simulink model "bee2_complex_corr"  (Simulink 7.0)
settings: Solver=ode45  StartTime=0.0  StopTime=10.0  RelTol=1e-3
undefined symbols (not defined in the file or in its folder): BEE2_usr
libraries: xbsIndex_r4 x279, xps_library x61, casper_library_misc x18
(part 1 of 4)
settings Model: Creator=Rurik A Primiani  LastModifiedBy=mdexter

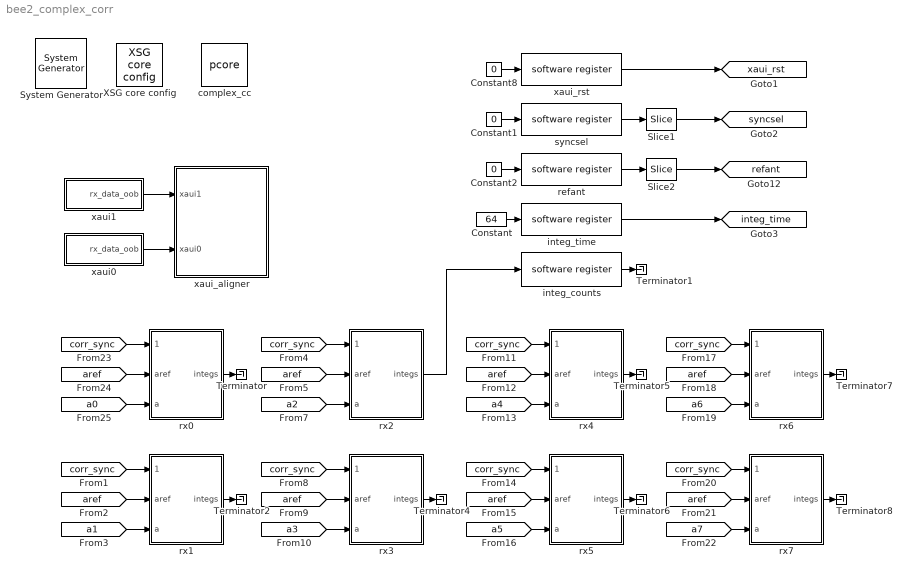
== system bee2_complex_corr ==
  " System Generator" : xbsIndex_r4/ System Generator  Tag=genX  SystemSampleTime=-1  xilinxfamily=virtex2p  part=xc2vp70  speed=-7  package=ff1704  synthesis_tool=XST  clock_wrapper=Clock Enables  directory=./bee2_complex_corr/sysgen  testbench=off  simulink_period=1  sysclk_period=3.9063  dcm_input_clock_period=100  incr_netlist=off  trim_vbits=Everywhere in SubSystem  dbl_ovrd=According to Block Masks  core_generation=According to Block Masks  run_coregen=off  deprecated_control=off  eval_field=0  block_type=sysgen
      settings: block_version=10.1.3
  Constant : Constant  Value=64
  Constant1 : Constant  Value=0
  Constant2 : Constant  Value=0
  Constant8 : Constant  Value=0
  Slice1 : xbsIndex_r4/Slice  nbits=2  boolean_output=off  mode=Lower Bit Location + Width  bit1=0  base1=MSB of Input  bit0=0  base0=LSB of Input  dbl_ovrd=off  block_type=slice
      settings: infoedit="Extracts a given range of bits from each input sample and presents it at the output.  The output type is ordinarily unsigned with binary point at zero, but can be Boolean when the slice is one bit wide.<P><P>Hardware notes: In hardware this block costs nothing."  block_version=10.1.3
  Slice2 : xbsIndex_r4/Slice  nbits=3  boolean_output=off  mode=Lower Bit Location + Width  bit1=0  base1=MSB of Input  bit0=0  base0=LSB of Input  dbl_ovrd=off  block_type=slice
      settings: infoedit="Extracts a given range of bits from each input sample and presents it at the output.  The output type is ordinarily unsigned with binary point at zero, but can be Boolean when the slice is one bit wide.<P><P>Hardware notes: In hardware this block costs nothing."  block_version=10.1.3
  Terminator{,1..2,4..8} (8 alike) : Terminator
  XSG core config : xps_library/XSG core config  Tag=xps:xsg  SystemSampleTime=-1  hw_sys=BEE2_usr  ibob_linux=off  clk_src=usr_clk2x  iBOB_clk_src=sys_clk  BEE2_ctrl_clk_src=sys_clk  BEE2_usr_clk_src=usr_clk2x  ROACH_clk_src=sys_clk  CORR_clk_src=sys_clk  gpio_clk_io_group=iBOB:sma  gpio_clk_bit_index=0  clk_rate=256  sample_period=1  synthesis_tool=XST  mpc_type=powerpc405
  complex_cc : xps_library/pcore  Tag=xps:pcore  SystemSampleTime=-1  pcore_path=complex_cc_core/complex_cc_core.ngc
  integ_counts : xps_library/software register  Tag=xps:sw_reg  SystemSampleTime=-1  io_dir=To Processor  arith_type=Unsigned  bitwidth=32  bin_pt=0  sample_period=1  gw_name=bee2_complex_corr_integ_counts_user_data_in
      link override convert: arith_type=Unsigned  n_bits=32  bin_pt=0
  integ_time : xps_library/software register  Tag=xps:sw_reg  SystemSampleTime=-1  io_dir=From Processor  arith_type=Unsigned  bitwidth=32  bin_pt=0  sample_period=1  gw_name=bee2_complex_corr_integ_time_user_data_out
      link override bee2_complex_corr_0x0_integ_time_user_data_out: arith_type=Unsigned  n_bits=32  bin_pt=0  period=1
      link override bee2_complex_corr_corr00_integ_time_user_data_out: arith_type=Unsigned  n_bits=32  bin_pt=0  period=1
      link override bee2_complex_corr_corr01_integ_time_user_data_out: arith_type=Unsigned  n_bits=32  bin_pt=0  period=1
      link override bee2_complex_corr_integ_time_user_data_out: arith_type=Unsigned  n_bits=32  bin_pt=0  period=1
      link override correlator_2bit_bee2_integ_time_user_data_out: arith_type=Unsigned  n_bits=32  bin_pt=0  period=1
      link override correlator_2bit_bee2_x2_integ_time_user_data_out: arith_type=Unsigned  n_bits=32  bin_pt=0  period=1
      link override correlator_2bit_ibob_integ_time_user_data_out: arith_type=Unsigned  n_bits=32  bin_pt=0  period=1
      link override dbe_xaui_corr_corr_integ_time_user_data_out: arith_type=Unsigned  n_bits=32  bin_pt=0  period=1
      link override dbe_xaui_corr_corr_integ_user_data_out: arith_type=Unsigned  n_bits=32  bin_pt=0  period=1
      link override dbe_xaui_corr_new_corr_integ_user_data_out: arith_type=Unsigned  n_bits=32  bin_pt=0  period=1
  refant : xps_library/software register  Tag=xps:sw_reg  SystemSampleTime=-1  io_dir=From Processor  arith_type=Unsigned  bitwidth=32  bin_pt=0  sample_period=1  gw_name=bee2_complex_corr_refant_user_data_out
      link override bee2_complex_corr_corr_rst_user_data_out: arith_type=Unsigned  n_bits=32  bin_pt=0  period=1
      link override bee2_complex_corr_refant_user_data_out: arith_type=Unsigned  n_bits=32  bin_pt=0  period=1
      link override correlator_2bit_bee2_integ_time_user_data_out: arith_type=Unsigned  n_bits=32  bin_pt=0  period=1
      link override correlator_2bit_bee2_x2_integ_time_user_data_out: arith_type=Unsigned  n_bits=32  bin_pt=0  period=1
      link override correlator_2bit_ibob_integ_time_user_data_out: arith_type=Unsigned  n_bits=32  bin_pt=0  period=1
      link override dbe_xaui_corr_corr_integ_user_data_out: arith_type=Unsigned  n_bits=32  bin_pt=0  period=1
      link override dbe_xaui_corr_corr_reset_user_data_out: arith_type=Unsigned  n_bits=32  bin_pt=0  period=1
      link override dbe_xaui_corr_new_corr_integ_user_data_out: arith_type=Unsigned  n_bits=32  bin_pt=0  period=1
  rx0 : Subsystem
  rx1 : Subsystem
  rx2 : Subsystem
  rx3 : Subsystem
  rx4 : Subsystem
  rx5 : Subsystem
  rx6 : Subsystem
  rx7 : Subsystem
  syncsel : xps_library/software register  Tag=xps:sw_reg  SystemSampleTime=-1  io_dir=From Processor  arith_type=Unsigned  bitwidth=32  bin_pt=0  sample_period=1  gw_name=bee2_complex_corr_syncsel_user_data_out
      link override bee2_complex_corr_corr_rst_user_data_out: arith_type=Unsigned  n_bits=32  bin_pt=0  period=1
      link override bee2_complex_corr_syncsel_user_data_out: arith_type=Unsigned  n_bits=32  bin_pt=0  period=1
      link override correlator_2bit_bee2_integ_time_user_data_out: arith_type=Unsigned  n_bits=32  bin_pt=0  period=1
      link override correlator_2bit_bee2_x2_integ_time_user_data_out: arith_type=Unsigned  n_bits=32  bin_pt=0  period=1
      link override correlator_2bit_ibob_integ_time_user_data_out: arith_type=Unsigned  n_bits=32  bin_pt=0  period=1
      link override dbe_xaui_corr_corr_integ_user_data_out: arith_type=Unsigned  n_bits=32  bin_pt=0  period=1
      link override dbe_xaui_corr_corr_reset_user_data_out: arith_type=Unsigned  n_bits=32  bin_pt=0  period=1
      link override dbe_xaui_corr_new_corr_integ_user_data_out: arith_type=Unsigned  n_bits=32  bin_pt=0  period=1
  xaui0 : Subsystem
  xaui1 : Subsystem
  xaui_aligner : Subsystem
  xaui_rst : xps_library/software register  Tag=xps:sw_reg  SystemSampleTime=-1  io_dir=From Processor  arith_type=Unsigned  bitwidth=32  bin_pt=0  sample_period=1  gw_name=bee2_complex_corr_xaui_rst_user_data_out
      link override bee2_complex_corr_xaui_rst_user_data_out: arith_type=Unsigned  n_bits=32  bin_pt=0  period=1
      link override dbe_xaui_corr_xaui_rst_user_data_out: arith_type=Unsigned  n_bits=32  bin_pt=0  period=1
      link override dbe_xaui_xaui_rst_user_data_out: arith_type=Unsigned  n_bits=32  bin_pt=0  period=1
      link override xaui_rx_reset_user_data_out: arith_type=Unsigned  n_bits=32  bin_pt=0  period=1
  tag scope: integ_time=global, refant=global, syncsel=global, xaui_rst=global
  wires:
  xaui1/1(rx_data_oob) -> xaui_aligner/1(xaui1)
  xaui0/1(rx_data_oob) -> xaui_aligner/2(xaui0)
  xaui_rst/1 -> [xaui_rst]
  Constant8/1 -> xaui_rst/1
  syncsel/1 -> Slice1/1
  Slice1/1 -> [syncsel]
  Constant1/1 -> syncsel/1
  [corr_sync] -> rx1/1(sync_in)
  [aref] -> rx1/2(aref)
  [a1] -> rx1/3(a)
  [corr_sync] -> rx2/1(sync_in)
  [aref] -> rx2/2(aref)
  [a2] -> rx2/3(a)
  [corr_sync] -> rx3/1(sync_in)
  [aref] -> rx3/2(aref)
  [a3] -> rx3/3(a)
  [corr_sync] -> rx4/1(sync_in)
  [aref] -> rx4/2(aref)
  [a4] -> rx4/3(a)
  [corr_sync] -> rx5/1(sync_in)
  [aref] -> rx5/2(aref)
  [a5] -> rx5/3(a)
  [corr_sync] -> rx6/1(sync_in)
  [aref] -> rx6/2(aref)
  [a6] -> rx6/3(a)
  [corr_sync] -> rx7/1(sync_in)
  [aref] -> rx7/2(aref)
  [a7] -> rx7/3(a)
  [corr_sync] -> rx0/1(sync_in)
  [aref] -> rx0/2(aref)
  [a0] -> rx0/3(a)
  refant/1 -> Slice2/1
  Slice2/1 -> [refant]
  Constant2/1 -> refant/1
  integ_time/1 -> [integ_time]
  rx0/1(integs) -> Terminator/1
  integ_counts/1 -> Terminator1/1
  Constant/1 -> integ_time/1
  rx1/1(integs) -> Terminator2/1
  rx3/1(integs) -> Terminator4/1
  rx4/1(integs) -> Terminator5/1
  rx5/1(integs) -> Terminator6/1
  rx6/1(integs) -> Terminator7/1
  rx7/1(integs) -> Terminator8/1
  rx2/1(integs) -> integ_counts/1

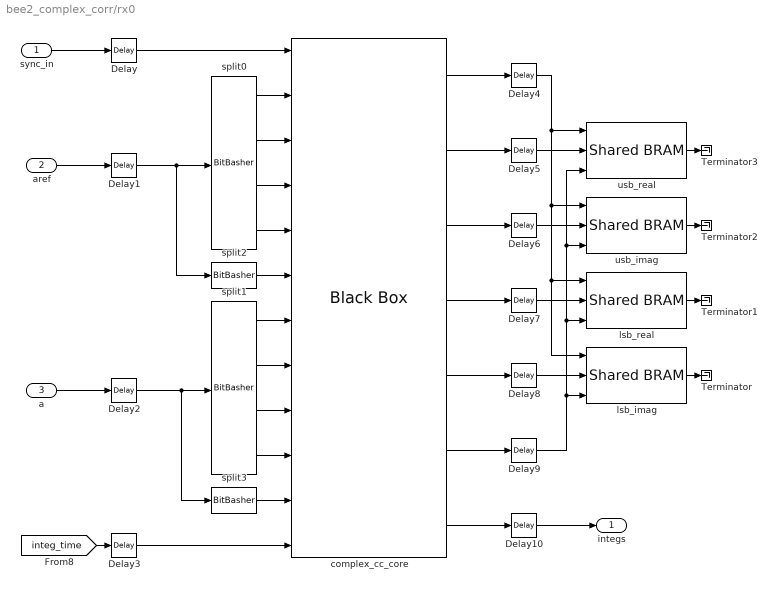
== system bee2_complex_corr/rx0 ==
  sync_in : Inport  OutDataType=sfix(16)  OutScaling=2^0
  aref : Inport  Port=2  OutDataType=sfix(16)  OutScaling=2^0
  a : Inport  Port=3  OutDataType=sfix(16)  OutScaling=2^0
  Delay{,1..10} (11 alike) : xbsIndex_r4/Delay  en=off  latency=1  dbl_ovrd=off  reg_retiming=off  block_type=delay
  Terminator{,1..3} (4 alike) : Terminator
  complex_cc_core : xbsIndex_r4/Black Box  init_code=complex_cc_core_config  sim_method=Inactive  block_type=blackbox2
      settings: infoedit="Incorporates black box HDL and simulation model into a System Generator design.<P><P>You must supply a Black Box with certain information about the HDL component you would like to bring into System Generator. This information is provided through a Matlab function.<P><P>When \"Simulation mode\" is set to \"Inactive\", you will typically want to provide a separate simulation model by using a Simulation Multiplexer.<P>When \"Simulation mode\" is set to \"External co-simulator\", you must include a ModelSim block in the design."  block_version=10.1.3
  lsb_imag : xps_library/Shared BRAM  Tag=xps:bram  SystemSampleTime=-1  arith_type="Signed  (2's comp)"  addr_width=11  data_width=32  data_bin_pt=0  init_vals=0  sample_rate=1
      link override bee2_complex_corr_0x0_func_real_data_out: arith_type="Signed  (2's comp)"
      link override bee2_complex_corr_corr00_func_real_data_out: arith_type="Signed  (2's comp)"
      link override bee2_complex_corr_corr01_func_real_data_out: arith_type="Signed  (2's comp)"
      link override bee2_complex_corr_rx0_lsb_imag_data_out: arith_type="Signed  (2's comp)"
      link override convert_din: arith_type="Signed  (2's comp)"
      link override correlator_2bit_bee2_output_corr0_data_out: arith_type=Unsigned
      link override correlator_2bit_bee2_x2_output_corr01_data_out: arith_type=Unsigned
      link override correlator_2bit_bee2_x2_output_corr0_data_out: arith_type=Unsigned
      link override correlator_2bit_ibob_output_corr0_data_out: arith_type=Unsigned
      link override cross_correlator_test_corr_out_data_out: arith_type="Signed  (2's comp)"
      link override cross_correlator_test_input_data1_data_out: arith_type=Unsigned
      link override dbe_xaui_corr_corr_func_data_out: arith_type="Signed  (2's comp)"
      link override dbe_xaui_corr_new_xaui_summer_summer_output_corr_data_out: arith_type="Signed  (2's comp)"
      link override dbe_xaui_corr_xaui_summer_summer_output_corr_data_out: arith_type="Signed  (2's comp)"
      link override mem/sim_data_in: arith_type="Signed  (2's comp)"
  lsb_real : xps_library/Shared BRAM  Tag=xps:bram  SystemSampleTime=-1  arith_type="Signed  (2's comp)"  addr_width=11  data_width=32  data_bin_pt=0  init_vals=0  sample_rate=1
      link override bee2_complex_corr_0x0_func_real_data_out: arith_type="Signed  (2's comp)"
      link override bee2_complex_corr_corr00_func_real_data_out: arith_type="Signed  (2's comp)"
      link override bee2_complex_corr_corr01_func_real_data_out: arith_type="Signed  (2's comp)"
      link override bee2_complex_corr_rx0_lsb_real_data_out: arith_type="Signed  (2's comp)"
      link override convert_din: arith_type="Signed  (2's comp)"
      link override correlator_2bit_bee2_output_corr0_data_out: arith_type=Unsigned
      link override correlator_2bit_bee2_x2_output_corr01_data_out: arith_type=Unsigned
      link override correlator_2bit_bee2_x2_output_corr0_data_out: arith_type=Unsigned
      link override correlator_2bit_ibob_output_corr0_data_out: arith_type=Unsigned
      link override cross_correlator_test_corr_out_data_out: arith_type="Signed  (2's comp)"
      link override cross_correlator_test_input_data1_data_out: arith_type=Unsigned
      link override dbe_xaui_corr_corr_func_data_out: arith_type="Signed  (2's comp)"
      link override dbe_xaui_corr_new_xaui_summer_summer_output_corr_data_out: arith_type="Signed  (2's comp)"
      link override dbe_xaui_corr_xaui_summer_summer_output_corr_data_out: arith_type="Signed  (2's comp)"
      link override mem/sim_data_in: arith_type="Signed  (2's comp)"
  split0 : xbsIndex_r4/BitBasher  bitexpr=|  display_expr=off  sr_1=1  arith_type1=Unsigned  bin_pt1=0  sr_2=2  arith_type2=Unsigned  bin_pt2=0  sr_3=3  arith_type3=Unsigned  bin_pt3=0  sr_4=4  arith_type4=Unsigned  bin_pt4=0  dbl_ovrd=off  block_type=bitbasher
      | <html><head><meta name="qrichtext" content="1" /><style type="text/css">
      | p, li { white-space: pre-wrap; }
      | </style></head><body style=" font-family:'MS Shell Dlg 2'; font-size:8.25pt; font-weight:400; font-style:normal;">
      | <p style=" margin-top:0px; margin-bottom:0px; margin-left:0px; margin-right:0px; -qt-block-indent:0; text-indent:0px; font-size:8pt;">r0={a[8:7]}<br />i0={a[6:5]}<br /><span style=" font-family:'MS Shell Dlg';">r1={a[4:3]}<br />i1={a[2:1]}</span></p></body></html>
      settings: block_version=10.1.3
  split1 : xbsIndex_r4/BitBasher  bitexpr=|  display_expr=off  sr_1=1  arith_type1=Unsigned  bin_pt1=0  sr_2=2  arith_type2=Unsigned  bin_pt2=0  sr_3=3  arith_type3=Unsigned  bin_pt3=0  sr_4=4  arith_type4=Unsigned  bin_pt4=0  dbl_ovrd=off  block_type=bitbasher
      | <html><head><meta name="qrichtext" content="1" /><style type="text/css">
      | p, li { white-space: pre-wrap; }
      | </style></head><body style=" font-family:'MS Shell Dlg 2'; font-size:8.25pt; font-weight:400; font-style:normal;">
      | <p style=" margin-top:0px; margin-bottom:0px; margin-left:0px; margin-right:0px; -qt-block-indent:0; text-indent:0px; font-size:8pt;">r0={a[8:7]}<br />i0={a[6:5]}<br /><span style=" font-family:'MS Shell Dlg';">r1={a[4:3]}<br />i1={a[2:1]}</span></p></body></html>
      settings: block_version=10.1.3
  split2 : xbsIndex_r4/BitBasher  bitexpr=|  display_expr=off  sr_1=1  arith_type1=Unsigned  bin_pt1=0  sr_2=2  arith_type2=Unsigned  bin_pt2=0  sr_3=3  arith_type3=Unsigned  bin_pt3=0  sr_4=4  arith_type4=Unsigned  bin_pt4=0  dbl_ovrd=off  block_type=bitbasher
      | <html><head><meta name="qrichtext" content="1" /><style type="text/css">
      | p, li { white-space: pre-wrap; }
      | </style></head><body style=" font-family:'MS Shell Dlg 2'; font-size:8.25pt; font-weight:400; font-style:normal;">
      | <p style=" margin-top:0px; margin-bottom:0px; margin-left:0px; margin-right:0px; -qt-block-indent:0; text-indent:0px; font-size:8pt;"><span style=" font-family:'MS Shell Dlg';">w={a[0]}</span></p></body></html>
      settings: block_version=10.1.3
  split3 : xbsIndex_r4/BitBasher  bitexpr=|  display_expr=off  sr_1=1  arith_type1=Unsigned  bin_pt1=0  sr_2=2  arith_type2=Unsigned  bin_pt2=0  sr_3=3  arith_type3=Unsigned  bin_pt3=0  sr_4=4  arith_type4=Unsigned  bin_pt4=0  dbl_ovrd=off  block_type=bitbasher
      | <html><head><meta name="qrichtext" content="1" /><style type="text/css">
      | p, li { white-space: pre-wrap; }
      | </style></head><body style=" font-family:'MS Shell Dlg 2'; font-size:8.25pt; font-weight:400; font-style:normal;">
      | <p style=" margin-top:0px; margin-bottom:0px; margin-left:0px; margin-right:0px; -qt-block-indent:0; text-indent:0px; font-size:8pt;"><span style=" font-family:'MS Shell Dlg';">w={a[0]}</span></p></body></html>
      settings: block_version=10.1.3
  usb_imag : xps_library/Shared BRAM  Tag=xps:bram  SystemSampleTime=-1  arith_type="Signed  (2's comp)"  addr_width=11  data_width=32  data_bin_pt=0  init_vals=0  sample_rate=1
      link override bee2_complex_corr_0x0_func_real_data_out: arith_type="Signed  (2's comp)"
      link override bee2_complex_corr_corr00_func_real_data_out: arith_type="Signed  (2's comp)"
      link override bee2_complex_corr_corr01_func_real_data_out: arith_type="Signed  (2's comp)"
      link override bee2_complex_corr_rx0_usb_imag_data_out: arith_type="Signed  (2's comp)"
      link override convert_din: arith_type="Signed  (2's comp)"
      link override correlator_2bit_bee2_output_corr0_data_out: arith_type=Unsigned
      link override correlator_2bit_bee2_x2_output_corr01_data_out: arith_type=Unsigned
      link override correlator_2bit_bee2_x2_output_corr0_data_out: arith_type=Unsigned
      link override correlator_2bit_ibob_output_corr0_data_out: arith_type=Unsigned
      link override cross_correlator_test_corr_out_data_out: arith_type="Signed  (2's comp)"
      link override cross_correlator_test_input_data1_data_out: arith_type=Unsigned
      link override dbe_xaui_corr_corr_func_data_out: arith_type="Signed  (2's comp)"
      link override dbe_xaui_corr_new_xaui_summer_summer_output_corr_data_out: arith_type="Signed  (2's comp)"
      link override dbe_xaui_corr_xaui_summer_summer_output_corr_data_out: arith_type="Signed  (2's comp)"
      link override mem/sim_data_in: arith_type="Signed  (2's comp)"
  usb_real : xps_library/Shared BRAM  Tag=xps:bram  SystemSampleTime=-1  arith_type="Signed  (2's comp)"  addr_width=11  data_width=32  data_bin_pt=0  init_vals=0  sample_rate=1
      link override bee2_complex_corr_0x0_func_real_data_out: arith_type="Signed  (2's comp)"
      link override bee2_complex_corr_corr00_func_real_data_out: arith_type="Signed  (2's comp)"
      link override bee2_complex_corr_corr01_func_real_data_out: arith_type="Signed  (2's comp)"
      link override bee2_complex_corr_rx0_usb_real_data_out: arith_type="Signed  (2's comp)"
      link override convert_din: arith_type="Signed  (2's comp)"
      link override correlator_2bit_bee2_output_corr0_data_out: arith_type=Unsigned
      link override correlator_2bit_bee2_x2_output_corr01_data_out: arith_type=Unsigned
      link override correlator_2bit_bee2_x2_output_corr0_data_out: arith_type=Unsigned
      link override correlator_2bit_ibob_output_corr0_data_out: arith_type=Unsigned
      link override cross_correlator_test_corr_out_data_out: arith_type="Signed  (2's comp)"
      link override cross_correlator_test_input_data1_data_out: arith_type=Unsigned
      link override dbe_xaui_corr_corr_func_data_out: arith_type="Signed  (2's comp)"
      link override dbe_xaui_corr_new_xaui_summer_summer_output_corr_data_out: arith_type="Signed  (2's comp)"
      link override dbe_xaui_corr_xaui_summer_summer_output_corr_data_out: arith_type="Signed  (2's comp)"
      link override mem/sim_data_in: arith_type="Signed  (2's comp)"
  integs : Outport  OutDataType=sfix(16)  OutScaling=2^0
  wires:
  [integ_time] -> Delay3/1
  a/1 -> Delay2/1
  aref/1 -> Delay1/1
  split0/4 -> complex_cc_core/5
  split0/3 -> complex_cc_core/4
  split0/2 -> complex_cc_core/3
  split0/1 -> complex_cc_core/2
  sync_in/1 -> Delay/1
  complex_cc_core/1 -> Delay4/1
  complex_cc_core/2 -> Delay5/1
  complex_cc_core/3 -> Delay6/1
  complex_cc_core/4 -> Delay7/1
  complex_cc_core/5 -> Delay8/1
  Delay/1 -> complex_cc_core/1
  Delay1/1 -> split0/1, split2/1
  Delay2/1 -> split1/1, split3/1
  Delay7/1 -> lsb_real/2
  Delay8/1 -> lsb_imag/2
  Delay10/1 -> integs/1
  complex_cc_core/6 -> Delay9/1
  complex_cc_core/7 -> Delay10/1
  Delay5/1 -> usb_real/2
  Delay6/1 -> usb_imag/2
  Delay3/1 -> complex_cc_core/12
  split2/1 -> complex_cc_core/6
  split1/1 -> complex_cc_core/7
  split1/2 -> complex_cc_core/8
  split1/3 -> complex_cc_core/9
  split1/4 -> complex_cc_core/10
  split3/1 -> complex_cc_core/11
  Delay4/1 -> usb_real/1, usb_imag/1, lsb_imag/1, lsb_real/1
  Delay9/1 -> usb_real/3, usb_imag/3, lsb_real/3, lsb_imag/3
  lsb_imag/1 -> Terminator/1
  lsb_real/1 -> Terminator1/1
  usb_imag/1 -> Terminator2/1
  usb_real/1 -> Terminator3/1

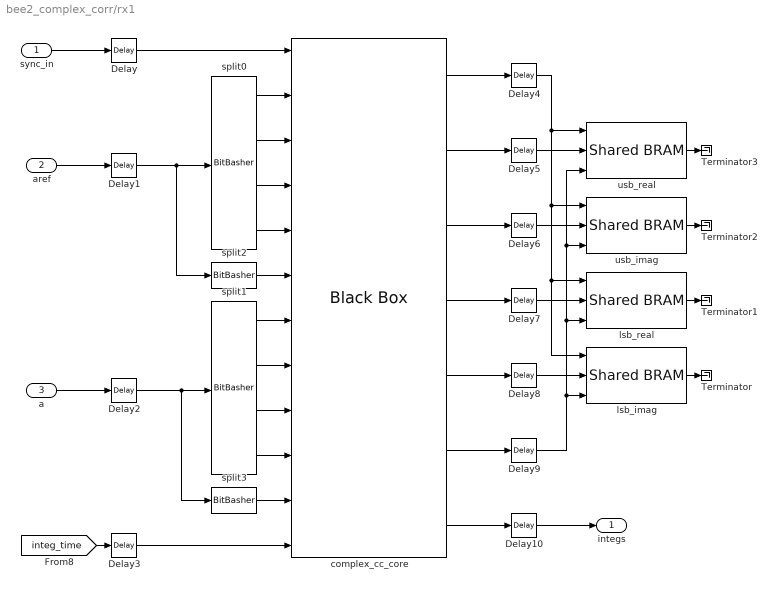
== system bee2_complex_corr/rx1 ==
  sync_in : Inport  OutDataType=sfix(16)  OutScaling=2^0
  aref : Inport  Port=2  OutDataType=sfix(16)  OutScaling=2^0
  a : Inport  Port=3  OutDataType=sfix(16)  OutScaling=2^0
  Delay{,1..10} (11 alike) : xbsIndex_r4/Delay  en=off  latency=1  dbl_ovrd=off  reg_retiming=off  block_type=delay
  Terminator{,1..3} (4 alike) : Terminator
  complex_cc_core : xbsIndex_r4/Black Box  init_code=complex_cc_core_config  sim_method=Inactive  block_type=blackbox2
      settings: infoedit="Incorporates black box HDL and simulation model into a System Generator design.<P><P>You must supply a Black Box with certain information about the HDL component you would like to bring into System Generator. This information is provided through a Matlab function.<P><P>When \"Simulation mode\" is set to \"Inactive\", you will typically want to provide a separate simulation model by using a Simulation Multiplexer.<P>When \"Simulation mode\" is set to \"External co-simulator\", you must include a ModelSim block in the design."  block_version=10.1.3
  lsb_imag : xps_library/Shared BRAM  Tag=xps:bram  SystemSampleTime=-1  arith_type="Signed  (2's comp)"  addr_width=11  data_width=32  data_bin_pt=0  init_vals=0  sample_rate=1
      link override bee2_complex_corr_0x0_func_real_data_out: arith_type="Signed  (2's comp)"
      link override bee2_complex_corr_corr00_func_real_data_out: arith_type="Signed  (2's comp)"
      link override bee2_complex_corr_corr01_func_real_data_out: arith_type="Signed  (2's comp)"
      link override bee2_complex_corr_rx1_lsb_imag_data_out: arith_type="Signed  (2's comp)"
      link override convert_din: arith_type="Signed  (2's comp)"
      link override correlator_2bit_bee2_output_corr0_data_out: arith_type=Unsigned
      link override correlator_2bit_bee2_x2_output_corr01_data_out: arith_type=Unsigned
      link override correlator_2bit_bee2_x2_output_corr0_data_out: arith_type=Unsigned
      link override correlator_2bit_ibob_output_corr0_data_out: arith_type=Unsigned
      link override cross_correlator_test_corr_out_data_out: arith_type="Signed  (2's comp)"
      link override cross_correlator_test_input_data1_data_out: arith_type=Unsigned
      link override dbe_xaui_corr_corr_func_data_out: arith_type="Signed  (2's comp)"
      link override dbe_xaui_corr_new_xaui_summer_summer_output_corr_data_out: arith_type="Signed  (2's comp)"
      link override dbe_xaui_corr_xaui_summer_summer_output_corr_data_out: arith_type="Signed  (2's comp)"
      link override mem/sim_data_in: arith_type="Signed  (2's comp)"
  lsb_real : xps_library/Shared BRAM  Tag=xps:bram  SystemSampleTime=-1  arith_type="Signed  (2's comp)"  addr_width=11  data_width=32  data_bin_pt=0  init_vals=0  sample_rate=1
      link override bee2_complex_corr_0x0_func_real_data_out: arith_type="Signed  (2's comp)"
      link override bee2_complex_corr_corr00_func_real_data_out: arith_type="Signed  (2's comp)"
      link override bee2_complex_corr_corr01_func_real_data_out: arith_type="Signed  (2's comp)"
      link override bee2_complex_corr_rx1_lsb_real_data_out: arith_type="Signed  (2's comp)"
      link override convert_din: arith_type="Signed  (2's comp)"
      link override correlator_2bit_bee2_output_corr0_data_out: arith_type=Unsigned
      link override correlator_2bit_bee2_x2_output_corr01_data_out: arith_type=Unsigned
      link override correlator_2bit_bee2_x2_output_corr0_data_out: arith_type=Unsigned
      link override correlator_2bit_ibob_output_corr0_data_out: arith_type=Unsigned
      link override cross_correlator_test_corr_out_data_out: arith_type="Signed  (2's comp)"
      link override cross_correlator_test_input_data1_data_out: arith_type=Unsigned
      link override dbe_xaui_corr_corr_func_data_out: arith_type="Signed  (2's comp)"
      link override dbe_xaui_corr_new_xaui_summer_summer_output_corr_data_out: arith_type="Signed  (2's comp)"
      link override dbe_xaui_corr_xaui_summer_summer_output_corr_data_out: arith_type="Signed  (2's comp)"
      link override mem/sim_data_in: arith_type="Signed  (2's comp)"
  split0 : xbsIndex_r4/BitBasher  bitexpr=|  display_expr=off  sr_1=1  arith_type1=Unsigned  bin_pt1=0  sr_2=2  arith_type2=Unsigned  bin_pt2=0  sr_3=3  arith_type3=Unsigned  bin_pt3=0  sr_4=4  arith_type4=Unsigned  bin_pt4=0  dbl_ovrd=off  block_type=bitbasher
      | <html><head><meta name="qrichtext" content="1" /><style type="text/css">
      | p, li { white-space: pre-wrap; }
      | </style></head><body style=" font-family:'MS Shell Dlg 2'; font-size:8.25pt; font-weight:400; font-style:normal;">
      | <p style=" margin-top:0px; margin-bottom:0px; margin-left:0px; margin-right:0px; -qt-block-indent:0; text-indent:0px; font-size:8pt;">r0={a[8:7]}<br />i0={a[6:5]}<br /><span style=" font-family:'MS Shell Dlg';">r1={a[4:3]}<br />i1={a[2:1]}</span></p></body></html>
      settings: block_version=10.1.3
  split1 : xbsIndex_r4/BitBasher  bitexpr=|  display_expr=off  sr_1=1  arith_type1=Unsigned  bin_pt1=0  sr_2=2  arith_type2=Unsigned  bin_pt2=0  sr_3=3  arith_type3=Unsigned  bin_pt3=0  sr_4=4  arith_type4=Unsigned  bin_pt4=0  dbl_ovrd=off  block_type=bitbasher
      | <html><head><meta name="qrichtext" content="1" /><style type="text/css">
      | p, li { white-space: pre-wrap; }
      | </style></head><body style=" font-family:'MS Shell Dlg 2'; font-size:8.25pt; font-weight:400; font-style:normal;">
      | <p style=" margin-top:0px; margin-bottom:0px; margin-left:0px; margin-right:0px; -qt-block-indent:0; text-indent:0px; font-size:8pt;">r0={a[8:7]}<br />i0={a[6:5]}<br /><span style=" font-family:'MS Shell Dlg';">r1={a[4:3]}<br />i1={a[2:1]}</span></p></body></html>
      settings: block_version=10.1.3
  split2 : xbsIndex_r4/BitBasher  bitexpr=|  display_expr=off  sr_1=1  arith_type1=Unsigned  bin_pt1=0  sr_2=2  arith_type2=Unsigned  bin_pt2=0  sr_3=3  arith_type3=Unsigned  bin_pt3=0  sr_4=4  arith_type4=Unsigned  bin_pt4=0  dbl_ovrd=off  block_type=bitbasher
      | <html><head><meta name="qrichtext" content="1" /><style type="text/css">
      | p, li { white-space: pre-wrap; }
      | </style></head><body style=" font-family:'MS Shell Dlg 2'; font-size:8.25pt; font-weight:400; font-style:normal;">
      | <p style=" margin-top:0px; margin-bottom:0px; margin-left:0px; margin-right:0px; -qt-block-indent:0; text-indent:0px; font-size:8pt;"><span style=" font-family:'MS Shell Dlg';">w={a[0]}</span></p></body></html>
      settings: block_version=10.1.3
  split3 : xbsIndex_r4/BitBasher  bitexpr=|  display_expr=off  sr_1=1  arith_type1=Unsigned  bin_pt1=0  sr_2=2  arith_type2=Unsigned  bin_pt2=0  sr_3=3  arith_type3=Unsigned  bin_pt3=0  sr_4=4  arith_type4=Unsigned  bin_pt4=0  dbl_ovrd=off  block_type=bitbasher
      | <html><head><meta name="qrichtext" content="1" /><style type="text/css">
      | p, li { white-space: pre-wrap; }
      | </style></head><body style=" font-family:'MS Shell Dlg 2'; font-size:8.25pt; font-weight:400; font-style:normal;">
      | <p style=" margin-top:0px; margin-bottom:0px; margin-left:0px; margin-right:0px; -qt-block-indent:0; text-indent:0px; font-size:8pt;"><span style=" font-family:'MS Shell Dlg';">w={a[0]}</span></p></body></html>
      settings: block_version=10.1.3
  usb_imag : xps_library/Shared BRAM  Tag=xps:bram  SystemSampleTime=-1  arith_type="Signed  (2's comp)"  addr_width=11  data_width=32  data_bin_pt=0  init_vals=0  sample_rate=1
      link override bee2_complex_corr_0x0_func_real_data_out: arith_type="Signed  (2's comp)"
      link override bee2_complex_corr_corr00_func_real_data_out: arith_type="Signed  (2's comp)"
      link override bee2_complex_corr_corr01_func_real_data_out: arith_type="Signed  (2's comp)"
      link override bee2_complex_corr_rx1_usb_imag_data_out: arith_type="Signed  (2's comp)"
      link override convert_din: arith_type="Signed  (2's comp)"
      link override correlator_2bit_bee2_output_corr0_data_out: arith_type=Unsigned
      link override correlator_2bit_bee2_x2_output_corr01_data_out: arith_type=Unsigned
      link override correlator_2bit_bee2_x2_output_corr0_data_out: arith_type=Unsigned
      link override correlator_2bit_ibob_output_corr0_data_out: arith_type=Unsigned
      link override cross_correlator_test_corr_out_data_out: arith_type="Signed  (2's comp)"
      link override cross_correlator_test_input_data1_data_out: arith_type=Unsigned
      link override dbe_xaui_corr_corr_func_data_out: arith_type="Signed  (2's comp)"
      link override dbe_xaui_corr_new_xaui_summer_summer_output_corr_data_out: arith_type="Signed  (2's comp)"
      link override dbe_xaui_corr_xaui_summer_summer_output_corr_data_out: arith_type="Signed  (2's comp)"
      link override mem/sim_data_in: arith_type="Signed  (2's comp)"
  usb_real : xps_library/Shared BRAM  Tag=xps:bram  SystemSampleTime=-1  arith_type="Signed  (2's comp)"  addr_width=11  data_width=32  data_bin_pt=0  init_vals=0  sample_rate=1
      link override bee2_complex_corr_0x0_func_real_data_out: arith_type="Signed  (2's comp)"
      link override bee2_complex_corr_corr00_func_real_data_out: arith_type="Signed  (2's comp)"
      link override bee2_complex_corr_corr01_func_real_data_out: arith_type="Signed  (2's comp)"
      link override bee2_complex_corr_rx1_usb_real_data_out: arith_type="Signed  (2's comp)"
      link override convert_din: arith_type="Signed  (2's comp)"
      link override correlator_2bit_bee2_output_corr0_data_out: arith_type=Unsigned
      link override correlator_2bit_bee2_x2_output_corr01_data_out: arith_type=Unsigned
      link override correlator_2bit_bee2_x2_output_corr0_data_out: arith_type=Unsigned
      link override correlator_2bit_ibob_output_corr0_data_out: arith_type=Unsigned
      link override cross_correlator_test_corr_out_data_out: arith_type="Signed  (2's comp)"
      link override cross_correlator_test_input_data1_data_out: arith_type=Unsigned
      link override dbe_xaui_corr_corr_func_data_out: arith_type="Signed  (2's comp)"
      link override dbe_xaui_corr_new_xaui_summer_summer_output_corr_data_out: arith_type="Signed  (2's comp)"
      link override dbe_xaui_corr_xaui_summer_summer_output_corr_data_out: arith_type="Signed  (2's comp)"
      link override mem/sim_data_in: arith_type="Signed  (2's comp)"
  integs : Outport  OutDataType=sfix(16)  OutScaling=2^0
  wires:
  [integ_time] -> Delay3/1
  a/1 -> Delay2/1
  aref/1 -> Delay1/1
  split0/4 -> complex_cc_core/5
  split0/3 -> complex_cc_core/4
  split0/2 -> complex_cc_core/3
  split0/1 -> complex_cc_core/2
  sync_in/1 -> Delay/1
  complex_cc_core/1 -> Delay4/1
  complex_cc_core/2 -> Delay5/1
  complex_cc_core/3 -> Delay6/1
  complex_cc_core/4 -> Delay7/1
  complex_cc_core/5 -> Delay8/1
  Delay/1 -> complex_cc_core/1
  Delay1/1 -> split0/1, split2/1
  Delay2/1 -> split1/1, split3/1
  Delay7/1 -> lsb_real/2
  Delay8/1 -> lsb_imag/2
  Delay10/1 -> integs/1
  complex_cc_core/6 -> Delay9/1
  complex_cc_core/7 -> Delay10/1
  Delay5/1 -> usb_real/2
  Delay6/1 -> usb_imag/2
  Delay3/1 -> complex_cc_core/12
  split2/1 -> complex_cc_core/6
  split1/1 -> complex_cc_core/7
  split1/2 -> complex_cc_core/8
  split1/3 -> complex_cc_core/9
  split1/4 -> complex_cc_core/10
  split3/1 -> complex_cc_core/11
  Delay4/1 -> usb_real/1, usb_imag/1, lsb_imag/1, lsb_real/1
  Delay9/1 -> usb_real/3, usb_imag/3, lsb_real/3, lsb_imag/3
  lsb_imag/1 -> Terminator/1
  lsb_real/1 -> Terminator1/1
  usb_imag/1 -> Terminator2/1
  usb_real/1 -> Terminator3/1

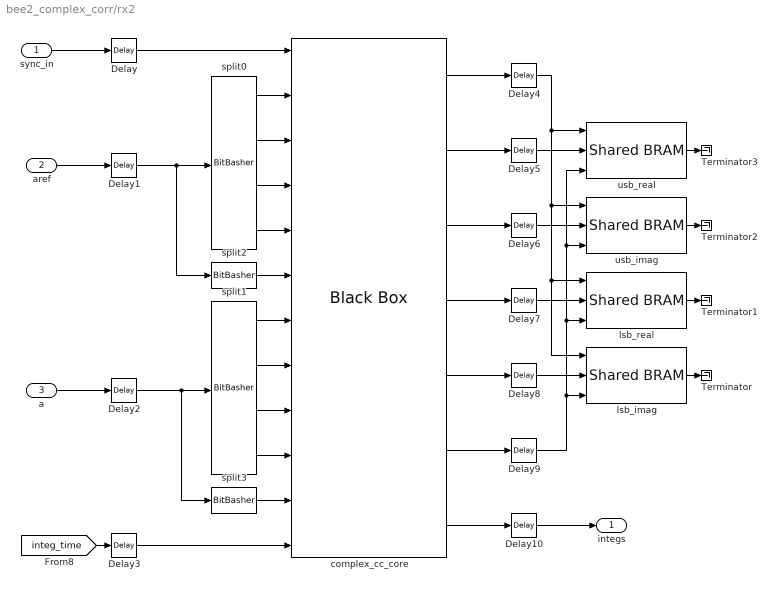
== system bee2_complex_corr/rx2 ==
  sync_in : Inport  OutDataType=sfix(16)  OutScaling=2^0
  aref : Inport  Port=2  OutDataType=sfix(16)  OutScaling=2^0
  a : Inport  Port=3  OutDataType=sfix(16)  OutScaling=2^0
  Delay{,1..10} (11 alike) : xbsIndex_r4/Delay  en=off  latency=1  dbl_ovrd=off  reg_retiming=off  block_type=delay
  Terminator{,1..3} (4 alike) : Terminator
  complex_cc_core : xbsIndex_r4/Black Box  init_code=complex_cc_core_config  sim_method=Inactive  block_type=blackbox2
      settings: infoedit="Incorporates black box HDL and simulation model into a System Generator design.<P><P>You must supply a Black Box with certain information about the HDL component you would like to bring into System Generator. This information is provided through a Matlab function.<P><P>When \"Simulation mode\" is set to \"Inactive\", you will typically want to provide a separate simulation model by using a Simulation Multiplexer.<P>When \"Simulation mode\" is set to \"External co-simulator\", you must include a ModelSim block in the design."  block_version=10.1.3
  lsb_imag : xps_library/Shared BRAM  Tag=xps:bram  SystemSampleTime=-1  arith_type="Signed  (2's comp)"  addr_width=11  data_width=32  data_bin_pt=0  init_vals=0  sample_rate=1
      link override bee2_complex_corr_0x0_func_real_data_out: arith_type="Signed  (2's comp)"
      link override bee2_complex_corr_corr00_func_real_data_out: arith_type="Signed  (2's comp)"
      link override bee2_complex_corr_corr01_func_real_data_out: arith_type="Signed  (2's comp)"
      link override bee2_complex_corr_rx2_lsb_imag_data_out: arith_type="Signed  (2's comp)"
      link override convert_din: arith_type="Signed  (2's comp)"
      link override correlator_2bit_bee2_output_corr0_data_out: arith_type=Unsigned
      link override correlator_2bit_bee2_x2_output_corr01_data_out: arith_type=Unsigned
      link override correlator_2bit_bee2_x2_output_corr0_data_out: arith_type=Unsigned
      link override correlator_2bit_ibob_output_corr0_data_out: arith_type=Unsigned
      link override cross_correlator_test_corr_out_data_out: arith_type="Signed  (2's comp)"
      link override cross_correlator_test_input_data1_data_out: arith_type=Unsigned
      link override dbe_xaui_corr_corr_func_data_out: arith_type="Signed  (2's comp)"
      link override dbe_xaui_corr_new_xaui_summer_summer_output_corr_data_out: arith_type="Signed  (2's comp)"
      link override dbe_xaui_corr_xaui_summer_summer_output_corr_data_out: arith_type="Signed  (2's comp)"
      link override mem/sim_data_in: arith_type="Signed  (2's comp)"
  lsb_real : xps_library/Shared BRAM  Tag=xps:bram  SystemSampleTime=-1  arith_type="Signed  (2's comp)"  addr_width=11  data_width=32  data_bin_pt=0  init_vals=0  sample_rate=1
      link override bee2_complex_corr_0x0_func_real_data_out: arith_type="Signed  (2's comp)"
      link override bee2_complex_corr_corr00_func_real_data_out: arith_type="Signed  (2's comp)"
      link override bee2_complex_corr_corr01_func_real_data_out: arith_type="Signed  (2's comp)"
      link override bee2_complex_corr_rx2_lsb_real_data_out: arith_type="Signed  (2's comp)"
      link override convert_din: arith_type="Signed  (2's comp)"
      link override correlator_2bit_bee2_output_corr0_data_out: arith_type=Unsigned
      link override correlator_2bit_bee2_x2_output_corr01_data_out: arith_type=Unsigned
      link override correlator_2bit_bee2_x2_output_corr0_data_out: arith_type=Unsigned
      link override correlator_2bit_ibob_output_corr0_data_out: arith_type=Unsigned
      link override cross_correlator_test_corr_out_data_out: arith_type="Signed  (2's comp)"
      link override cross_correlator_test_input_data1_data_out: arith_type=Unsigned
      link override dbe_xaui_corr_corr_func_data_out: arith_type="Signed  (2's comp)"
      link override dbe_xaui_corr_new_xaui_summer_summer_output_corr_data_out: arith_type="Signed  (2's comp)"
      link override dbe_xaui_corr_xaui_summer_summer_output_corr_data_out: arith_type="Signed  (2's comp)"
      link override mem/sim_data_in: arith_type="Signed  (2's comp)"
  split0 : xbsIndex_r4/BitBasher  bitexpr=|  display_expr=off  sr_1=1  arith_type1=Unsigned  bin_pt1=0  sr_2=2  arith_type2=Unsigned  bin_pt2=0  sr_3=3  arith_type3=Unsigned  bin_pt3=0  sr_4=4  arith_type4=Unsigned  bin_pt4=0  dbl_ovrd=off  block_type=bitbasher
      | <html><head><meta name="qrichtext" content="1" /><style type="text/css">
      | p, li { white-space: pre-wrap; }
      | </style></head><body style=" font-family:'MS Shell Dlg 2'; font-size:8.25pt; font-weight:400; font-style:normal;">
      | <p style=" margin-top:0px; margin-bottom:0px; margin-left:0px; margin-right:0px; -qt-block-indent:0; text-indent:0px; font-size:8pt;">r0={a[8:7]}<br />i0={a[6:5]}<br /><span style=" font-family:'MS Shell Dlg';">r1={a[4:3]}<br />i1={a[2:1]}</span></p></body></html>
      settings: block_version=10.1.3
  split1 : xbsIndex_r4/BitBasher  bitexpr=|  display_expr=off  sr_1=1  arith_type1=Unsigned  bin_pt1=0  sr_2=2  arith_type2=Unsigned  bin_pt2=0  sr_3=3  arith_type3=Unsigned  bin_pt3=0  sr_4=4  arith_type4=Unsigned  bin_pt4=0  dbl_ovrd=off  block_type=bitbasher
      | <html><head><meta name="qrichtext" content="1" /><style type="text/css">
      | p, li { white-space: pre-wrap; }
      | </style></head><body style=" font-family:'MS Shell Dlg 2'; font-size:8.25pt; font-weight:400; font-style:normal;">
      | <p style=" margin-top:0px; margin-bottom:0px; margin-left:0px; margin-right:0px; -qt-block-indent:0; text-indent:0px; font-size:8pt;">r0={a[8:7]}<br />i0={a[6:5]}<br /><span style=" font-family:'MS Shell Dlg';">r1={a[4:3]}<br />i1={a[2:1]}</span></p></body></html>
      settings: block_version=10.1.3
  split2 : xbsIndex_r4/BitBasher  bitexpr=|  display_expr=off  sr_1=1  arith_type1=Unsigned  bin_pt1=0  sr_2=2  arith_type2=Unsigned  bin_pt2=0  sr_3=3  arith_type3=Unsigned  bin_pt3=0  sr_4=4  arith_type4=Unsigned  bin_pt4=0  dbl_ovrd=off  block_type=bitbasher
      | <html><head><meta name="qrichtext" content="1" /><style type="text/css">
      | p, li { white-space: pre-wrap; }
      | </style></head><body style=" font-family:'MS Shell Dlg 2'; font-size:8.25pt; font-weight:400; font-style:normal;">
      | <p style=" margin-top:0px; margin-bottom:0px; margin-left:0px; margin-right:0px; -qt-block-indent:0; text-indent:0px; font-size:8pt;"><span style=" font-family:'MS Shell Dlg';">w={a[0]}</span></p></body></html>
      settings: block_version=10.1.3
  split3 : xbsIndex_r4/BitBasher  bitexpr=|  display_expr=off  sr_1=1  arith_type1=Unsigned  bin_pt1=0  sr_2=2  arith_type2=Unsigned  bin_pt2=0  sr_3=3  arith_type3=Unsigned  bin_pt3=0  sr_4=4  arith_type4=Unsigned  bin_pt4=0  dbl_ovrd=off  block_type=bitbasher
      | <html><head><meta name="qrichtext" content="1" /><style type="text/css">
      | p, li { white-space: pre-wrap; }
      | </style></head><body style=" font-family:'MS Shell Dlg 2'; font-size:8.25pt; font-weight:400; font-style:normal;">
      | <p style=" margin-top:0px; margin-bottom:0px; margin-left:0px; margin-right:0px; -qt-block-indent:0; text-indent:0px; font-size:8pt;"><span style=" font-family:'MS Shell Dlg';">w={a[0]}</span></p></body></html>
      settings: block_version=10.1.3
  usb_imag : xps_library/Shared BRAM  Tag=xps:bram  SystemSampleTime=-1  arith_type="Signed  (2's comp)"  addr_width=11  data_width=32  data_bin_pt=0  init_vals=0  sample_rate=1
      link override bee2_complex_corr_0x0_func_real_data_out: arith_type="Signed  (2's comp)"
      link override bee2_complex_corr_corr00_func_real_data_out: arith_type="Signed  (2's comp)"
      link override bee2_complex_corr_corr01_func_real_data_out: arith_type="Signed  (2's comp)"
      link override bee2_complex_corr_rx2_usb_imag_data_out: arith_type="Signed  (2's comp)"
      link override convert_din: arith_type="Signed  (2's comp)"
      link override correlator_2bit_bee2_output_corr0_data_out: arith_type=Unsigned
      link override correlator_2bit_bee2_x2_output_corr01_data_out: arith_type=Unsigned
      link override correlator_2bit_bee2_x2_output_corr0_data_out: arith_type=Unsigned
      link override correlator_2bit_ibob_output_corr0_data_out: arith_type=Unsigned
      link override cross_correlator_test_corr_out_data_out: arith_type="Signed  (2's comp)"
      link override cross_correlator_test_input_data1_data_out: arith_type=Unsigned
      link override dbe_xaui_corr_corr_func_data_out: arith_type="Signed  (2's comp)"
      link override dbe_xaui_corr_new_xaui_summer_summer_output_corr_data_out: arith_type="Signed  (2's comp)"
      link override dbe_xaui_corr_xaui_summer_summer_output_corr_data_out: arith_type="Signed  (2's comp)"
      link override mem/sim_data_in: arith_type="Signed  (2's comp)"
  usb_real : xps_library/Shared BRAM  Tag=xps:bram  SystemSampleTime=-1  arith_type="Signed  (2's comp)"  addr_width=11  data_width=32  data_bin_pt=0  init_vals=0  sample_rate=1
      link override bee2_complex_corr_0x0_func_real_data_out: arith_type="Signed  (2's comp)"
      link override bee2_complex_corr_corr00_func_real_data_out: arith_type="Signed  (2's comp)"
      link override bee2_complex_corr_corr01_func_real_data_out: arith_type="Signed  (2's comp)"
      link override bee2_complex_corr_rx2_usb_real_data_out: arith_type="Signed  (2's comp)"
      link override convert_din: arith_type="Signed  (2's comp)"
      link override correlator_2bit_bee2_output_corr0_data_out: arith_type=Unsigned
      link override correlator_2bit_bee2_x2_output_corr01_data_out: arith_type=Unsigned
      link override correlator_2bit_bee2_x2_output_corr0_data_out: arith_type=Unsigned
      link override correlator_2bit_ibob_output_corr0_data_out: arith_type=Unsigned
      link override cross_correlator_test_corr_out_data_out: arith_type="Signed  (2's comp)"
      link override cross_correlator_test_input_data1_data_out: arith_type=Unsigned
      link override dbe_xaui_corr_corr_func_data_out: arith_type="Signed  (2's comp)"
      link override dbe_xaui_corr_new_xaui_summer_summer_output_corr_data_out: arith_type="Signed  (2's comp)"
      link override dbe_xaui_corr_xaui_summer_summer_output_corr_data_out: arith_type="Signed  (2's comp)"
      link override mem/sim_data_in: arith_type="Signed  (2's comp)"
  integs : Outport  OutDataType=sfix(16)  OutScaling=2^0
  wires:
  [integ_time] -> Delay3/1
  a/1 -> Delay2/1
  aref/1 -> Delay1/1
  split0/4 -> complex_cc_core/5
  split0/3 -> complex_cc_core/4
  split0/2 -> complex_cc_core/3
  split0/1 -> complex_cc_core/2
  sync_in/1 -> Delay/1
  complex_cc_core/1 -> Delay4/1
  complex_cc_core/2 -> Delay5/1
  complex_cc_core/3 -> Delay6/1
  complex_cc_core/4 -> Delay7/1
  complex_cc_core/5 -> Delay8/1
  Delay/1 -> complex_cc_core/1
  Delay1/1 -> split0/1, split2/1
  Delay2/1 -> split1/1, split3/1
  Delay7/1 -> lsb_real/2
  Delay8/1 -> lsb_imag/2
  Delay10/1 -> integs/1
  complex_cc_core/6 -> Delay9/1
  complex_cc_core/7 -> Delay10/1
  Delay5/1 -> usb_real/2
  Delay6/1 -> usb_imag/2
  Delay3/1 -> complex_cc_core/12
  split2/1 -> complex_cc_core/6
  split1/1 -> complex_cc_core/7
  split1/2 -> complex_cc_core/8
  split1/3 -> complex_cc_core/9
  split1/4 -> complex_cc_core/10
  split3/1 -> complex_cc_core/11
  Delay4/1 -> usb_real/1, usb_imag/1, lsb_imag/1, lsb_real/1
  Delay9/1 -> usb_real/3, usb_imag/3, lsb_real/3, lsb_imag/3
  lsb_imag/1 -> Terminator/1
  lsb_real/1 -> Terminator1/1
  usb_imag/1 -> Terminator2/1
  usb_real/1 -> Terminator3/1
